simulink model "test_mdl_gw"  (R2018a)
settings: Solver=VariableStepAuto  StartTime=0.0  StopTime=10.0  RelTol=1e-3
(part 2 of 2)

== system test_mdl_gw/BrakeSysFeatures_2/TRLR_SWAY_EVNT_IN_PROG ==
  in : Inport
  out : Outport
  wires:
  in/1 -> out/1

== system test_mdl_gw/BrakeSysFeatures_3/AirDamUp_B_RqBrk ==
  in : Inport
  out : Outport
  wires:
  in/1 -> out/1

== system test_mdl_gw/BrakeSysFeatures_3/ApaBrk_D_Stat ==
  in : Inport
  out : Outport
  wires:
  in/1 -> out/1

== system test_mdl_gw/BrakeSysFeatures_3/AutoHoldMde_D_Ind ==
  in : Inport
  out : Outport
  wires:
  in/1 -> out/1

== system test_mdl_gw/BrakeSysFeatures_3/AutoHoldMsgTxt_D_Rq ==
  in : Inport
  out : Outport
  wires:
  in/1 -> out/1

== system test_mdl_gw/BrakeSysFeatures_3/AutoHoldSwMde_B_Ind ==
  in : Inport
  out : Outport
  wires:
  in/1 -> out/1

== system test_mdl_gw/BrakeSysFeatures_3/BrkBstrVac_D_Stat ==
  in : Inport
  out : Outport
  wires:
  in/1 -> out/1

== system test_mdl_gw/BrakeSysFeatures_3/CtaBrk_D_Stat ==
  in : Inport
  out : Outport
  wires:
  in/1 -> out/1

== system test_mdl_gw/BrakeSysFeatures_3/DrvSlipCtlMdeMsg_D_Rq ==
  in : Inport
  out : Outport
  wires:
  in/1 -> out/1

== system test_mdl_gw/BrakeSysFeatures_3/DrvSlipCtlOffLamp_D_Rq ==
  in : Inport
  out : Outport
  wires:
  in/1 -> out/1

== system test_mdl_gw/BrakeSysFeatures_3/RbaBrk_D_Stat ==
  in : Inport
  out : Outport
  wires:
  in/1 -> out/1

== system test_mdl_gw/BrakeSysFeatures_3/SelDrvMdeAwd_D_Rq ==
  in : Inport
  out : Outport
  wires:
  in/1 -> out/1

== system test_mdl_gw/BrakeSysFeatures_3/SelDrvMdeChassis2_D_Rq ==
  in : Inport
  out : Outport
  wires:
  in/1 -> out/1

== system test_mdl_gw/BrakeSysFeatures_3/SelDrvMdeChassis_D_Rq ==
  in : Inport
  out : Outport
  wires:
  in/1 -> out/1

== system test_mdl_gw/BrakeSysFeatures_3/TrailCtlMsgTxt_D_Rq ==
  in : Inport
  out : Outport
  wires:
  in/1 -> out/1

== system test_mdl_gw/BrakeSysFeatures_3/TrailCtl_D_Stat ==
  in : Inport
  out : Outport
  wires:
  in/1 -> out/1

== system test_mdl_gw/DesiredTorqBrk/AbsActv_B_Actl ==
  in : Inport
  out : Outport
  wires:
  in/1 -> out/1

== system test_mdl_gw/DesiredTorqBrk/AccBrkActv_B_Actl ==
  in : Inport
  out : Outport
  wires:
  in/1 -> out/1

== system test_mdl_gw/DesiredTorqBrk/AccBrkDeny_B_Actl ==
  in : Inport
  out : Outport
  wires:
  in/1 -> out/1

== system test_mdl_gw/DesiredTorqBrk/AccBrkDis_B_Actl ==
  in : Inport
  out : Outport
  wires:
  in/1 -> out/1

== system test_mdl_gw/DesiredTorqBrk/AccBrkPrchgActv_B_Actl ==
  in : Inport
  out : Outport
  wires:
  in/1 -> out/1

== system test_mdl_gw/DesiredTorqBrk/AccBrkTotTqMn_B_Actl ==
  in : Inport
  out : Outport
  wires:
  in/1 -> out/1

== system test_mdl_gw/DesiredTorqBrk/AccBrkWarm_B_Actl ==
  in : Inport
  out : Outport
  wires:
  in/1 -> out/1

== system test_mdl_gw/DesiredTorqBrk/AccDis_B_ActlEpb ==
  in : Inport
  out : Outport
  wires:
  in/1 -> out/1

== system test_mdl_gw/DesiredTorqBrk/AccStopActv_B_ActlBrk ==
  in : Inport
  out : Outport
  wires:
  in/1 -> out/1

== system test_mdl_gw/DesiredTorqBrk/CcDis_B_Cmd ==
  in : Inport
  out : Outport
  wires:
  in/1 -> out/1

== system test_mdl_gw/DesiredTorqBrk/CmbbBaSensInc_B_Actl ==
  in : Inport
  out : Outport
  wires:
  in/1 -> out/1

== system test_mdl_gw/DesiredTorqBrk/CmbbBrkDecel_B_Actl ==
  in : Inport
  out : Outport
  wires:
  in/1 -> out/1

== system test_mdl_gw/DesiredTorqBrk/CmbbBrkDis_B_Actl ==
  in : Inport
  out : Outport
  wires:
  in/1 -> out/1

== system test_mdl_gw/DesiredTorqBrk/CmbbBrkPrchg_B_Actl ==
  in : Inport
  out : Outport
  wires:
  in/1 -> out/1

== system test_mdl_gw/DesiredTorqBrk/CmbbDeny_B_ActlBrk ==
  in : Inport
  out : Outport
  wires:
  in/1 -> out/1

== system test_mdl_gw/DesiredTorqBrk/LscmbBrkPrchg_B_Actl ==
  in : Inport
  out : Outport
  wires:
  in/1 -> out/1

== system test_mdl_gw/DesiredTorqBrk/LscmbbBaSensInc_B_Actl ==
  in : Inport
  out : Outport
  wires:
  in/1 -> out/1

== system test_mdl_gw/DesiredTorqBrk/LscmbbBrkDecel_B_Actl ==
  in : Inport
  out : Outport
  wires:
  in/1 -> out/1

== system test_mdl_gw/DesiredTorqBrk/LscmbbBrkDis_B_Actl ==
  in : Inport
  out : Outport
  wires:
  in/1 -> out/1

== system test_mdl_gw/DesiredTorqBrk/LscmbbDeny_B_ActlBrk ==
  in : Inport
  out : Outport
  wires:
  in/1 -> out/1

== system test_mdl_gw/DesiredTorqBrk/LscmbbMntr_B_Err ==
  in : Inport
  out : Outport
  wires:
  in/1 -> out/1

== system test_mdl_gw/DesiredTorqBrk/PrkBrkMsgTxt_D_Rq ==
  in : Inport
  out : Outport
  wires:
  in/1 -> out/1

== system test_mdl_gw/DesiredTorqBrk/PrkBrkRedLamp_D_Rq ==
  in : Inport
  out : Outport
  wires:
  in/1 -> out/1

== system test_mdl_gw/DesiredTorqBrk/PrkBrkStatus ==
  in : Inport
  out : Outport
  wires:
  in/1 -> out/1

== system test_mdl_gw/DesiredTorqBrk/PrkBrkYwLamp_D_Rq ==
  in : Inport
  out : Outport
  wires:
  in/1 -> out/1

== system test_mdl_gw/DesiredTorqBrk/PrplDrgCtlActv_B_Actl ==
  in : Inport
  out : Outport
  wires:
  in/1 -> out/1

== system test_mdl_gw/DesiredTorqBrk/PrplWhlTot_Tq_RqMx ==
  in : Inport
  out : Outport
  wires:
  in/1 -> out/1

== system test_mdl_gw/DesiredTorqBrk/StabCtlBrkActv_B_Actl ==
  in : Inport
  out : Outport
  wires:
  in/1 -> out/1

== system test_mdl_gw/DesiredTorqBrk/TracCtlPtActv_B_Actl ==
  in : Inport
  out : Outport
  wires:
  in/1 -> out/1

== system test_mdl_gw/DesiredTorqBrk/VehLongOvrGnd_A_Est ==
  in : Inport
  out : Outport
  wires:
  in/1 -> out/1

== system test_mdl_gw/DesiredTorqBrk/VehStop_D_Stat ==
  in : Inport
  out : Outport
  wires:
  in/1 -> out/1

== system test_mdl_gw/DesiredTorqBrk_2/PrplWhlTot_Tq_RqMn ==
  in : Inport
  out : Outport
  wires:
  in/1 -> out/1

== system test_mdl_gw/DesiredTorqBrk_2/PrplWhlTqRqMn_No_Cnt ==
  in : Inport
  out : Outport
  wires:
  in/1 -> out/1

== system test_mdl_gw/DesiredTorqBrk_2/PrplWhlTqRqMn_No_Cs ==
  in : Inport
  out : Outport
  wires:
  in/1 -> out/1

== system test_mdl_gw/DesiredTorqBrk_2/RgenBrkDynoMde_B_Actl ==
  in : Inport
  out : Outport
  wires:
  in/1 -> out/1

== system test_mdl_gw/DesiredTorqBrk_2/RgenTqFalt_B_Actl ==
  in : Inport
  out : Outport
  wires:
  in/1 -> out/1

== system test_mdl_gw/Global_PATS_SubTarget/immoSubTarget1Cmd_T1 ==
  in : Inport
  out : Outport
  wires:
  in/1 -> out/1

== system test_mdl_gw/Global_PATS_SubTarget/immoSubTarget1Data_T1 ==
  in : Inport
  out : Outport
  wires:
  in/1 -> out/1

== system test_mdl_gw/OTAPhysABStoGWM_ECG/OTAPhysABStoGWM_ECG ==
  in : Inport
  out : Outport
  wires:
  in/1 -> out/1

== system test_mdl_gw/PARSEDPhysABStoGWM_ECG/PARSEDPhysABStoGWM_ECG ==
  in : Inport
  out : Outport
  wires:
  in/1 -> out/1

== system test_mdl_gw/PARSEDPushABStoGWM_ECG/PARSEDPhysABS2toGWM_ECG ==
  in : Inport
  out : Outport
  wires:
  in/1 -> out/1

== system test_mdl_gw/SelectDriveModeData/ActvDrvMde_D2_Stat ==
  in : Inport
  out : Outport
  wires:
  in/1 -> out/1

== system test_mdl_gw/SelectDriveModeData/AutoEpbButtnOn_B_Stat ==
  in : Inport
  out : Outport
  wires:
  in/1 -> out/1

== system test_mdl_gw/SelectDriveModeData/AutoEpbDsply_D_Stat ==
  in : Inport
  out : Outport
  wires:
  in/1 -> out/1

== system test_mdl_gw/SelectDriveModeData/AutoEpbMsgTxt_D_Rq ==
  in : Inport
  out : Outport
  wires:
  in/1 -> out/1

== system test_mdl_gw/SelectDriveModeData/AwdMde_D_RqBrk ==
  in : Inport
  out : Outport
  wires:
  in/1 -> out/1

== system test_mdl_gw/SelectDriveModeData/SelDrvMdeMsgTxt_D_Rq ==
  in : Inport
  out : Outport
  wires:
  in/1 -> out/1

== system test_mdl_gw/SelectDriveModeData/SelDrvMdePos01_B_Avail ==
  in : Inport
  out : Outport
  wires:
  in/1 -> out/1

== system test_mdl_gw/SelectDriveModeData/SelDrvMdePos02_B_Avail ==
  in : Inport
  out : Outport
  wires:
  in/1 -> out/1

== system test_mdl_gw/SelectDriveModeData/SelDrvMdePos03_B_Avail ==
  in : Inport
  out : Outport
  wires:
  in/1 -> out/1

== system test_mdl_gw/SelectDriveModeData/SelDrvMdePos04_B_Avail ==
  in : Inport
  out : Outport
  wires:
  in/1 -> out/1

== system test_mdl_gw/SelectDriveModeData/SelDrvMdePos05_B_Avail ==
  in : Inport
  out : Outport
  wires:
  in/1 -> out/1

== system test_mdl_gw/SelectDriveModeData/SelDrvMdePos06_B_Avail ==
  in : Inport
  out : Outport
  wires:
  in/1 -> out/1

== system test_mdl_gw/SelectDriveModeData/SelDrvMdePos07_B_Avail ==
  in : Inport
  out : Outport
  wires:
  in/1 -> out/1

== system test_mdl_gw/SelectDriveModeData/SelDrvMdePos08_B_Avail ==
  in : Inport
  out : Outport
  wires:
  in/1 -> out/1

== system test_mdl_gw/SelectDriveModeData/SelDrvMdePos09_B_Avail ==
  in : Inport
  out : Outport
  wires:
  in/1 -> out/1

== system test_mdl_gw/SelectDriveModeData/SelDrvMdePos10_B_Avail ==
  in : Inport
  out : Outport
  wires:
  in/1 -> out/1

== system test_mdl_gw/SelectDriveModeData/SelDrvMdePos11_B_Avail ==
  in : Inport
  out : Outport
  wires:
  in/1 -> out/1

== system test_mdl_gw/SelectDriveModeData/SelDrvMdePos12_B_Avail ==
  in : Inport
  out : Outport
  wires:
  in/1 -> out/1

== system test_mdl_gw/SelectDriveModeData/SelDrvMdePt_D_Rq ==
  in : Inport
  out : Outport
  wires:
  in/1 -> out/1

== system test_mdl_gw/SelectDriveModeData/SelDrvMde_D2_Rq ==
  in : Inport
  out : Outport
  wires:
  in/1 -> out/1

== system test_mdl_gw/SelectDriveModeData/SelDrvMde_D_Stat ==
  in : Inport
  out : Outport
  wires:
  in/1 -> out/1

== system test_mdl_gw/SelectDriveModeData2/SelDrvMdePos01_D_Stat ==
  in : Inport
  out : Outport
  wires:
  in/1 -> out/1

== system test_mdl_gw/SelectDriveModeData2/SelDrvMdePos02_D_Stat ==
  in : Inport
  out : Outport
  wires:
  in/1 -> out/1

== system test_mdl_gw/SelectDriveModeData2/SelDrvMdePos03_D_Stat ==
  in : Inport
  out : Outport
  wires:
  in/1 -> out/1

== system test_mdl_gw/SelectDriveModeData2/SelDrvMdePos04_D_Stat ==
  in : Inport
  out : Outport
  wires:
  in/1 -> out/1

== system test_mdl_gw/SelectDriveModeData2/SelDrvMdePos05_D_Stat ==
  in : Inport
  out : Outport
  wires:
  in/1 -> out/1

== system test_mdl_gw/SelectDriveModeData2/SelDrvMdePos06_D_Stat ==
  in : Inport
  out : Outport
  wires:
  in/1 -> out/1

== system test_mdl_gw/SelectDriveModeData2/SelDrvMdePos07_D_Stat ==
  in : Inport
  out : Outport
  wires:
  in/1 -> out/1

== system test_mdl_gw/SelectDriveModeData2/SelDrvMdePos08_D_Stat ==
  in : Inport
  out : Outport
  wires:
  in/1 -> out/1

== system test_mdl_gw/SelectDriveModeData2/SelDrvMdePos09_D_Stat ==
  in : Inport
  out : Outport
  wires:
  in/1 -> out/1

== system test_mdl_gw/SelectDriveModeData2/SelDrvMdePos10_D_Stat ==
  in : Inport
  out : Outport
  wires:
  in/1 -> out/1

== system test_mdl_gw/SelectDriveModeData2/SelDrvMdePos11_D_Stat ==
  in : Inport
  out : Outport
  wires:
  in/1 -> out/1

== system test_mdl_gw/SelectDriveModeData2/SelDrvMdePos12_D_Stat ==
  in : Inport
  out : Outport
  wires:
  in/1 -> out/1

== system test_mdl_gw/TesterPhysicalResABS/TesterPhysicalResABS ==
  in : Inport
  out : Outport
  wires:
  in/1 -> out/1

== system test_mdl_gw/TrailerBrakeData/TrlrBrk_Pc_Rq ==
  in : Inport
  out : Outport
  wires:
  in/1 -> out/1

== system test_mdl_gw/TrailerBrakeData/VehPtch_An_Dsply ==
  in : Inport
  out : Outport
  wires:
  in/1 -> out/1

== system test_mdl_gw/TrailerBrakeData/VehRol_An_Dsply ==
  in : Inport
  out : Outport
  wires:
  in/1 -> out/1

== system test_mdl_gw/WheelData/BrkObdData_No_Actl ==
  in : Inport
  out : Outport
  wires:
  in/1 -> out/1

== system test_mdl_gw/WheelData/BrkObdIndex_No_Actl ==
  in : Inport
  out : Outport
  wires:
  in/1 -> out/1

== system test_mdl_gw/WheelData/WhlDirFl_D_Actl ==
  in : Inport
  out : Outport
  wires:
  in/1 -> out/1

== system test_mdl_gw/WheelData/WhlDirFr_D_Actl ==
  in : Inport
  out : Outport
  wires:
  in/1 -> out/1

== system test_mdl_gw/WheelData/WhlDirRl_D_Actl ==
  in : Inport
  out : Outport
  wires:
  in/1 -> out/1

== system test_mdl_gw/WheelData/WhlDirRr_D_Actl ==
  in : Inport
  out : Outport
  wires:
  in/1 -> out/1

== system test_mdl_gw/WheelData/WhlRotatFl_No_Cnt ==
  in : Inport
  out : Outport
  wires:
  in/1 -> out/1

== system test_mdl_gw/WheelData/WhlRotatFr_No_Cnt ==
  in : Inport
  out : Outport
  wires:
  in/1 -> out/1

== system test_mdl_gw/WheelData/WhlRotatRl_No_Cnt ==
  in : Inport
  out : Outport
  wires:
  in/1 -> out/1

== system test_mdl_gw/WheelData/WhlRotatRr_No_Cnt ==
  in : Inport
  out : Outport
  wires:
  in/1 -> out/1

== system test_mdl_gw/WheelSpeed/WhlFl_W_Meas ==
  in : Inport
  out : Outport
  wires:
  in/1 -> out/1

== system test_mdl_gw/WheelSpeed/WhlFr_W_Meas ==
  in : Inport
  out : Outport
  wires:
  in/1 -> out/1

== system test_mdl_gw/WheelSpeed/WhlRl_W_Meas ==
  in : Inport
  out : Outport
  wires:
  in/1 -> out/1

== system test_mdl_gw/WheelSpeed/WhlRr_W_Meas ==
  in : Inport
  out : Outport
  wires:
  in/1 -> out/1
